simulink model "colorednoise_sim"  (Simulink 8.6)
settings: Solver=ode45  StartTime=0.0  StopTime=10.0  RelTol=1e-3
settings Model: Creator=mgilson  LastModifiedBy=hgarnier  ExtModeAutoUpdateStatusClock=off
settings OptimizationCC: InitFltsAndDblsToZero=on
settings DebuggingCC: SaveWithParameterizedLinksMsg=none  FcnCallInpInsideContextMsg=UseLocalSettings  StrictBusMsg=Warning
settings GRTTargetCC: TargetFcnLib=ansi_tfl_tmw.mat  GeneratePreprocessorConditionals=Use local settings

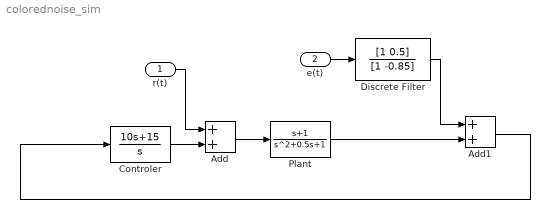
== system colorednoise_sim ==
  r(t) : Inport
  e(t) : Inport  Port=2
  Add : Sum
  Add1 : Sum
  Controler : TransferFcn  Numerator=[10 15]  Denominator=[1 0]
  Discrete Filter : DiscreteFilter  Numerator=[1 0.5]  Denominator=[1 -0.85]  SampleTime=1
  Plant : TransferFcn  Numerator=[1 1]  Denominator="[1  0.5 1]"
  wires:
  Controler/1 -> Add/2
  Add/1 -> Plant/1
  Plant/1 -> Add1/2
  Add1/1 -> Controler/1
  r(t)/1 -> Add/1
  Discrete Filter/1 -> Add1/1
  e(t)/1 -> Discrete Filter/1
